simulink model "SNAP_Simulink_model_vtest"  (R2020b)
settings: Solver=VariableStepAuto  StartTime=0.0  StopTime=SNAP_sim_length  FixedStep=0.1  MaxStep=10  RelTol=1e-4  EnableMultiTasking=on
InitFcn:
  | SNAP_Simulink_Init_Function
undefined symbols (not defined in the file or in its folder): aeroCIP2006, EN_2BodyModel, EN_Aero, EN_GG, EN_Hyst, EN_Mag, initial_position, initial_velocity, magnitude, SNAP_Br, SNAP_Bs, SNAP_CONST_a3H0, SNAP_CONST_earth_mag_dipole, SNAP_CONST_G_earth, SNAP_CONST_m_earth, SNAP_CONST_mu0, SNAP_CONST_r_earth, SNAP_Hc, SNAP_init_rates, SNAP_JD, SNAP_magnets, SNAP_sat_inertia, SNAP_sat_mass, SNAP_starting_ECI2ECEF_dcm, SNAP_V_hyst, SNAPaero
libraries: vrlib x22, aerolibtransform2 x8, simulink x6, aerolibconvert2 x5, aerolibobsolete x1, aerolibanim x1
(part 2 of 2)

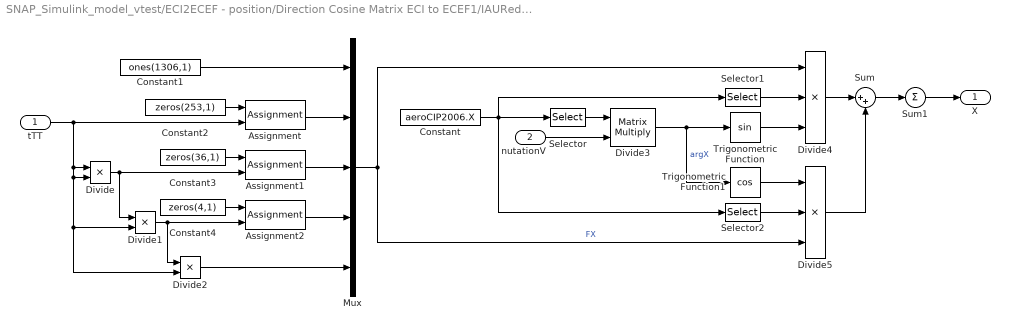
== system SNAP_Simulink_model_vtest/ECI2ECEF - position/Direction Cosine Matrix ECI to ECEF1/IAUReduction/Celestial motion of the CIP/P03 Precession/X ==
  tTT : Inport
  nutationV : Inport  Port=2
  Assignment : Assignment  IndexOptions=Assign all  Indices=1  OutputSizes=1
  Assignment1 : Assignment  IndexOptions=Assign all  Indices=1  OutputSizes=1
  Assignment2 : Assignment  IndexOptions=Assign all  Indices=1  OutputSizes=1
  Constant : Constant  Value=aeroCIP2006.X
  Constant1 : Constant  Value=ones(1306,1)
  Constant2 : Constant  Value=zeros(253,1)
  Constant3 : Constant  Value=zeros(36,1)
  Constant4 : Constant  Value=zeros(4,1)
  Divide : Product  Inputs=**
  Divide1 : Product  Inputs=**
  Divide2 : Product  Inputs=**
  Divide3 : Product  Inputs=**  Multiplication=Matrix(*)
  Divide4 : Product  Inputs=***
  Divide5 : Product  Inputs=***
  Mux : Mux  Inputs=5
  Selector : Selector  NumberOfDimensions=2  InputPortWidth=3  IndexOptions=Select all,Starting index (dialog)  Indices=[1 3],4  OutputSizes=1,14
  Selector1 : Selector  NumberOfDimensions=2  InputPortWidth=3  IndexOptions=Select all,Index vector (dialog)  Indices=[1 3],2  OutputSizes=1,14
  Selector2 : Selector  NumberOfDimensions=2  InputPortWidth=3  IndexOptions=Select all,Index vector (dialog)  Indices=[1 3],3  OutputSizes=1,14
  Sum : Sum  Inputs=|++
  Sum1 : Sum  Inputs=|+|
  Trigonometric Function : Trigonometry
  Trigonometric Function1 : Trigonometry  Operator=cos
  X : Outport
  wires:
  Constant1/1 -> Mux/1
  Assignment/1 -> Mux/2
  Assignment1/1 -> Mux/3
  Assignment2/1 -> Mux/4
  Divide2/1 -> Mux/5
  Sum1/1 -> X/1
  Sum/1 -> Sum1/1
  Divide5/1 -> Sum/2
  Divide4/1 -> Sum/1
  Mux/1 -> Divide5/3, Divide4/1  "FX"
  Selector2/1 -> Divide5/2
  Trigonometric Function1/1 -> Divide5/1
  Selector1/1 -> Divide4/2
  Trigonometric Function/1 -> Divide4/3
  Divide3/1 -> Trigonometric Function/1, Trigonometric Function1/1  "argX"
  Selector/1 -> Divide3/1
  nutationV/1 -> Divide3/2
  Constant/1 -> Selector/1, Selector1/1, Selector2/1
  Divide/1 -> Assignment1/2, Divide1/1
  Divide1/1 -> Assignment2/2, Divide2/1
  Constant4/1 -> Assignment2/1
  Constant3/1 -> Assignment1/1
  tTT/1 -> Divide/1, Divide/2, Divide1/2, Divide2/2, Assignment/2
  Constant2/1 -> Assignment/1

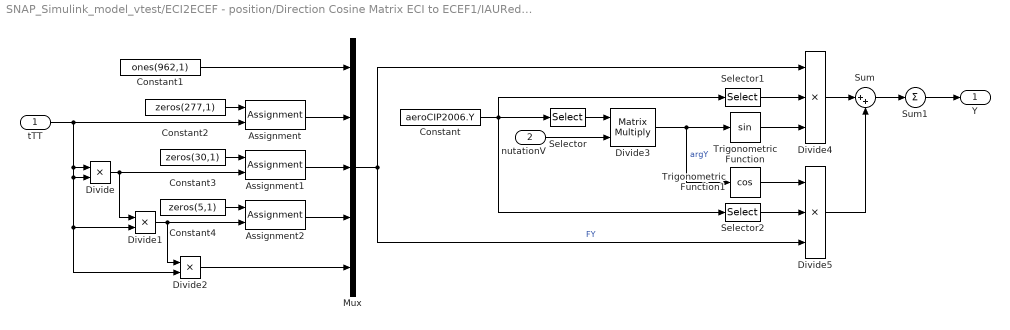
== system SNAP_Simulink_model_vtest/ECI2ECEF - position/Direction Cosine Matrix ECI to ECEF1/IAUReduction/Celestial motion of the CIP/P03 Precession/Y ==
  tTT : Inport
  nutationV : Inport  Port=2
  Assignment : Assignment  IndexOptions=Assign all  Indices=1  OutputSizes=1
  Assignment1 : Assignment  IndexOptions=Assign all  Indices=1  OutputSizes=1
  Assignment2 : Assignment  IndexOptions=Assign all  Indices=1  OutputSizes=1
  Constant : Constant  Value=aeroCIP2006.Y
  Constant1 : Constant  Value=ones(962,1)
  Constant2 : Constant  Value=zeros(277,1)
  Constant3 : Constant  Value=zeros(30,1)
  Constant4 : Constant  Value=zeros(5,1)
  Divide : Product  Inputs=**
  Divide1 : Product  Inputs=**
  Divide2 : Product  Inputs=**
  Divide3 : Product  Inputs=**  Multiplication=Matrix(*)
  Divide4 : Product  Inputs=***
  Divide5 : Product  Inputs=***
  Mux : Mux  Inputs=5
  Selector : Selector  NumberOfDimensions=2  InputPortWidth=3  IndexOptions=Select all,Starting index (dialog)  Indices=[1 3],4  OutputSizes=1,14
  Selector1 : Selector  NumberOfDimensions=2  InputPortWidth=3  IndexOptions=Select all,Index vector (dialog)  Indices=[1 3],2  OutputSizes=1,14
  Selector2 : Selector  NumberOfDimensions=2  InputPortWidth=3  IndexOptions=Select all,Index vector (dialog)  Indices=[1 3],3  OutputSizes=1,14
  Sum : Sum  Inputs=|++
  Sum1 : Sum  Inputs=|+|
  Trigonometric Function : Trigonometry
  Trigonometric Function1 : Trigonometry  Operator=cos
  Y : Outport
  wires:
  Constant2/1 -> Assignment/1
  tTT/1 -> Assignment/2, Divide2/2, Divide1/2, Divide/2, Divide/1
  Constant3/1 -> Assignment1/1
  Constant4/1 -> Assignment2/1
  Divide1/1 -> Divide2/1, Assignment2/2
  Divide/1 -> Divide1/1, Assignment1/2
  Constant/1 -> Selector2/1, Selector1/1, Selector/1
  nutationV/1 -> Divide3/2
  Selector/1 -> Divide3/1
  Divide3/1 -> Trigonometric Function1/1, Trigonometric Function/1  "argY"
  Trigonometric Function/1 -> Divide4/3
  Selector1/1 -> Divide4/2
  Trigonometric Function1/1 -> Divide5/1
  Selector2/1 -> Divide5/2
  Mux/1 -> Divide4/1, Divide5/3  "FY"
  Divide4/1 -> Sum/1
  Divide5/1 -> Sum/2
  Sum/1 -> Sum1/1
  Sum1/1 -> Y/1
  Divide2/1 -> Mux/5
  Assignment2/1 -> Mux/4
  Assignment1/1 -> Mux/3
  Assignment/1 -> Mux/2
  Constant1/1 -> Mux/1

== matlab function SNAP_Simulink_model_vtest/Hysteresis Material/Hysteresis Curve Model/Hysteresis Model ==
  data: B input; DBDT output; H input; DHDT input; Bsx input; Brx input; Hcx input
function DBDT = fcn(B, H, DHDT, Bsx, Brx, Hcx)
%#eml
mu0 = 4*pi*1e-7; 
% Bsx = 0.73 * 1e4;  %Tesla
% Brx = 0.35 * 1e4;
% Hcx = 1.59;  %A/m

k = 0.6;
p = 4.75;
q0 = 0.0885;

HL = tan(pi.*B./2./Bsx)./k - Hcx;

BP = 2 .* k .* Bsx/pi .* cos(pi*B/2/Bsx)*2;

F = (H-HL)/2/Hcx;

% neg = find(DHDT<0);
% F(neg) = 1-F(neg);

for i =1:3
    if(DHDT(i)<0)
        F(i) = 1-F(i);
    end
end


Q = q0 + (1-q0).*F.*p;

DBDT = Q.*BP.*DHDT;

% Based on this paper:
% "A MAGNETIC HYSTERESIS MODEL", Thomas W. Flatley, 1995
% http://ntrs.nasa.gov/archive/nasa/casi.ntrs.nasa.gov/19950021380_1995121380.pdf
